simulink model "Control_Logic_e"  (R2021a)
settings: Solver=FixedStepAuto  StartTime=Start_time  StopTime=Stop_time  FixedStep=Sample_time  RelTol=1e-3
undefined symbols (not defined in the file or in its folder): Aset_N1, Aset_N10, Aset_N11, Aset_N12, Aset_N2, Aset_N3, Aset_N4, Aset_N5, Aset_N6, Aset_N7, Aset_N8, Aset_N9, Dset_N1, Dset_N2, Sample_time
(part 3 of 3)

== matlab function Control_Logic_e/OSHOTC8/OSHOTC ==
  data: u input; y output; old input; w_old input
% ワンショット タイマ
%  xがOFFからONに変化してからパラメータで設定した[sec]の間、yをONとする。
%  なお、xのON状態がパラメータで設定した[sec]以上継続した場合、あるいは設定以下
%  しか継続しない場合でも、yのON状態の期間はパラメータで設定した時間となる。
%       ud(1) = u(1) ;:入力信号
%       yold = u(2) ;:前回値
%       set = u(3) ;:時定数
%       timc(1) = u(4) ;:計算刻み
%       timc(2) = u(5) ;:経過時間
%       y : 出力信号
function y  = OSHOTC(u,old,w_old)
       y = zeros(2,1);
       ud1 = logical(u(1));
       yold = logical(old(1));
       set = u(2);
       timc1 = u(3);
       timc2 = w_old(1);
       
    if (ud1 == false) && (yold == false)
        w = 0;
        temp = false;
    else
        if set > timc2
            temp = true;
            w = timc2 + timc1;
        else
            temp = false;
            w = timc2;
            if ud1 == false
                w = 0;
            end
        end
    end
    y(1) = double(temp);
    y(2) = w;
end

== matlab function Control_Logic_e/OSHOTC11/OSHOTC ==
  data: u input; y output; old input; w_old input
% ワンショット タイマ
%  xがOFFからONに変化してからパラメータで設定した[sec]の間、yをONとする。
%  なお、xのON状態がパラメータで設定した[sec]以上継続した場合、あるいは設定以下
%  しか継続しない場合でも、yのON状態の期間はパラメータで設定した時間となる。
%       ud(1) = u(1) ;:入力信号
%       yold = u(2) ;:前回値
%       set = u(3) ;:時定数
%       timc(1) = u(4) ;:計算刻み
%       timc(2) = u(5) ;:経過時間
%       y : 出力信号
function y  = OSHOTC(u,old,w_old)
       y = zeros(2,1);
       ud1 = logical(u(1));
       yold = logical(old(1));
       set = u(2);
       timc1 = u(3);
       timc2 = w_old(1);
       
    if (ud1 == false) && (yold == false)
        w = 0;
        temp = false;
    else
        if set > timc2
            temp = true;
            w = timc2 + timc1;
        else
            temp = false;
            w = timc2;
            if ud1 == false
                w = 0;
            end
        end
    end
    y(1) = double(temp);
    y(2) = w;
end

== matlab function Control_Logic_e/OSHOTC13/OSHOTC ==
  data: u input; y output; old input; w_old input
% ワンショット タイマ
%  xがOFFからONに変化してからパラメータで設定した[sec]の間、yをONとする。
%  なお、xのON状態がパラメータで設定した[sec]以上継続した場合、あるいは設定以下
%  しか継続しない場合でも、yのON状態の期間はパラメータで設定した時間となる。
%       ud(1) = u(1) ;:入力信号
%       yold = u(2) ;:前回値
%       set = u(3) ;:時定数
%       timc(1) = u(4) ;:計算刻み
%       timc(2) = u(5) ;:経過時間
%       y : 出力信号
function y  = OSHOTC(u,old,w_old)
       y = zeros(2,1);
       ud1 = logical(u(1));
       yold = logical(old(1));
       set = u(2);
       timc1 = u(3);
       timc2 = w_old(1);
       
    if (ud1 == false) && (yold == false)
        w = 0;
        temp = false;
    else
        if set > timc2
            temp = true;
            w = timc2 + timc1;
        else
            temp = false;
            w = timc2;
            if ud1 == false
                w = 0;
            end
        end
    end
    y(1) = double(temp);
    y(2) = w;
end

== matlab function Control_Logic_e/NOT4/NOT ==
  data: u input; y output
%反転
function y  = NOT(u)
    y = 0;
    ud = logical(u(1));
    if ud == false        
        temp = true;
    else
        temp = false;
    end
    y = double(temp);
end

== matlab function Control_Logic_e/OSHOTC6/OSHOTC ==
  data: u input; y output; old input; w_old input
% ワンショット タイマ
%  xがOFFからONに変化してからパラメータで設定した[sec]の間、yをONとする。
%  なお、xのON状態がパラメータで設定した[sec]以上継続した場合、あるいは設定以下
%  しか継続しない場合でも、yのON状態の期間はパラメータで設定した時間となる。
%       ud(1) = u(1) ;:入力信号
%       yold = u(2) ;:前回値
%       set = u(3) ;:時定数
%       timc(1) = u(4) ;:計算刻み
%       timc(2) = u(5) ;:経過時間
%       y : 出力信号
function y  = OSHOTC(u,old,w_old)
       y = zeros(2,1);
       ud1 = logical(u(1));
       yold = logical(old(1));
       set = u(2);
       timc1 = u(3);
       timc2 = w_old(1);
       
    if (ud1 == false) && (yold == false)
        w = 0;
        temp = false;
    else
        if set > timc2
            temp = true;
            w = timc2 + timc1;
        else
            temp = false;
            w = timc2;
            if ud1 == false
                w = 0;
            end
        end
    end
    y(1) = double(temp);
    y(2) = w;
end

== matlab function Control_Logic_e/OSHOTC7/OSHOTC ==
  data: u input; y output; old input; w_old input
% ワンショット タイマ
%  xがOFFからONに変化してからパラメータで設定した[sec]の間、yをONとする。
%  なお、xのON状態がパラメータで設定した[sec]以上継続した場合、あるいは設定以下
%  しか継続しない場合でも、yのON状態の期間はパラメータで設定した時間となる。
%       ud(1) = u(1) ;:入力信号
%       yold = u(2) ;:前回値
%       set = u(3) ;:時定数
%       timc(1) = u(4) ;:計算刻み
%       timc(2) = u(5) ;:経過時間
%       y : 出力信号
function y  = OSHOTC(u,old,w_old)
       y = zeros(2,1);
       ud1 = logical(u(1));
       yold = logical(old(1));
       set = u(2);
       timc1 = u(3);
       timc2 = w_old(1);
       
    if (ud1 == false) && (yold == false)
        w = 0;
        temp = false;
    else
        if set > timc2
            temp = true;
            w = timc2 + timc1;
        else
            temp = false;
            w = timc2;
            if ud1 == false
                w = 0;
            end
        end
    end
    y(1) = double(temp);
    y(2) = w;
end

== matlab function Control_Logic_e/OSHOTC14/OSHOTC ==
  data: u input; y output; old input; w_old input
% ワンショット タイマ
%  xがOFFからONに変化してからパラメータで設定した[sec]の間、yをONとする。
%  なお、xのON状態がパラメータで設定した[sec]以上継続した場合、あるいは設定以下
%  しか継続しない場合でも、yのON状態の期間はパラメータで設定した時間となる。
%       ud(1) = u(1) ;:入力信号
%       yold = u(2) ;:前回値
%       set = u(3) ;:時定数
%       timc(1) = u(4) ;:計算刻み
%       timc(2) = u(5) ;:経過時間
%       y : 出力信号
function y  = OSHOTC(u,old,w_old)
       y = zeros(2,1);
       ud1 = logical(u(1));
       yold = logical(old(1));
       set = u(2);
       timc1 = u(3);
       timc2 = w_old(1);
       
    if (ud1 == false) && (yold == false)
        w = 0;
        temp = false;
    else
        if set > timc2
            temp = true;
            w = timc2 + timc1;
        else
            temp = false;
            w = timc2;
            if ud1 == false
                w = 0;
            end
        end
    end
    y(1) = double(temp);
    y(2) = w;
end

== matlab function Control_Logic_e/OR4/MATLAB Function ==
  data: u input; y output
% 論理積
function y  = OR(u)
   y= 0;
   dy = false;
   for i = 1:size(u,1)
   dy = logical(u(i)) | dy;
   end
    y = double(dy);
end

== matlab function Control_Logic_e/OR3/MATLAB Function ==
  data: u input; y output
% 論理積
function y  = OR(u)
   y= 0;
   dy = false;
   for i = 1:size(u,1)
   dy = logical(u(i)) | dy;
   end
    y = double(dy);
end

== matlab function Control_Logic_e/OR5/MATLAB Function ==
  data: u input; y output
% 論理積
function y  = OR(u)
   y= 0;
   dy = false;
   for i = 1:size(u,1)
   dy = logical(u(i)) | dy;
   end
    y = double(dy);
end

== matlab function Control_Logic_e/OR6/MATLAB Function ==
  data: u input; y output
% 論理積
function y  = OR(u)
   y= 0;
   dy = false;
   for i = 1:size(u,1)
   dy = logical(u(i)) | dy;
   end
    y = double(dy);
end

== matlab function Control_Logic_e/OR/MATLAB Function ==
  data: u input; y output
% 論理積
function y  = OR(u)
   y= 0;
   dy = false;
   for i = 1:size(u,1)
   dy = logical(u(i)) | dy;
   end
    y = double(dy);
end

== matlab function Control_Logic_e/OR8/MATLAB Function ==
  data: u input; y output
% 論理積
function y  = OR(u)
   y= 0;
   dy = false;
   for i = 1:size(u,1)
   dy = logical(u(i)) | dy;
   end
    y = double(dy);
end

== matlab function Control_Logic_e/NOT5/NOT ==
  data: u input; y output
%反転
function y  = NOT(u)
    y = 0;
    ud = logical(u(1));
    if ud == false        
        temp = true;
    else
        temp = false;
    end
    y = double(temp);
end

== matlab function Control_Logic_e/OR9/MATLAB Function ==
  data: u input; y output
% 論理積
function y  = OR(u)
   y= 0;
   dy = false;
   for i = 1:size(u,1)
   dy = logical(u(i)) | dy;
   end
    y = double(dy);
end

== matlab function Control_Logic_e/OR7/MATLAB Function ==
  data: u input; y output
% 論理積
function y  = OR(u)
   y= 0;
   dy = false;
   for i = 1:size(u,1)
   dy = logical(u(i)) | dy;
   end
    y = double(dy);
end

== matlab function Control_Logic_e/OR1/MATLAB Function ==
  data: u input; y output
% 論理積
function y  = OR(u)
   y= 0;
   dy = false;
   for i = 1:size(u,1)
   dy = logical(u(i)) | dy;
   end
    y = double(dy);
end

== matlab function Control_Logic_e/ANSW6/MATLAB Function ==
  data: u input; y output
% 2位置(アナログ)スイッチ
%   u3入力がONならば、 y=x1(A入力を選択)
%   u3入力がOFFならば、 y=x2(B入力を選択)
%       u(2):A入力変数
%       u(3):B入力変数
%       u3=u(1):C入力変数
%       y : 出力変数
function y  = ANSW(u)
    y = 0;
    temp = logical(u(1));
    temp2 = 0;
    if temp ~= false
        temp2 = u(2);
    else
        temp2 = u(3); 
    end
    y = temp2;
end

== matlab function Control_Logic_e/LAG/LAG ==
  data: u input; y output; old input
%% lag 1次遅れ
%   function:		PLAG
%    description:	一次遅れ
%	y=(dt×x+τ×yold)/(dt+τ)
%	dt：時間刻み，τ：時定数，yold：前回出力値
%
%    algorithm:
%	if(init == TRUE)	then
%		AY = Y_old = AX
%	endif
%	AY = (dt*AX+τ*Y_old)/(dt+ τ)
%	Y_old = AY

function y  = LAG(u,old)
  y = 0;
  x = u(1);
  tau = u(2);
  dt = u(3);
  y_old = old(1);
  y = (dt*x+tau*y_old)/(dt+ tau);
end

== matlab function Control_Logic_e/LAG1/LAG ==
  data: u input; y output; old input
%% lag 1次遅れ
%   function:		PLAG
%    description:	一次遅れ
%	y=(dt×x+τ×yold)/(dt+τ)
%	dt：時間刻み，τ：時定数，yold：前回出力値
%
%    algorithm:
%	if(init == TRUE)	then
%		AY = Y_old = AX
%	endif
%	AY = (dt*AX+τ*Y_old)/(dt+ τ)
%	Y_old = AY

function y  = LAG(u,old)
  y = 0;
  x = u(1);
  tau = u(2);
  dt = u(3);
  y_old = old(1);
  y = (dt*x+tau*y_old)/(dt+ tau);
end

== matlab function Control_Logic_e/LAG2/LAG ==
  data: u input; y output; old input
%% lag 1次遅れ
%   function:		PLAG
%    description:	一次遅れ
%	y=(dt×x+τ×yold)/(dt+τ)
%	dt：時間刻み，τ：時定数，yold：前回出力値
%
%    algorithm:
%	if(init == TRUE)	then
%		AY = Y_old = AX
%	endif
%	AY = (dt*AX+τ*Y_old)/(dt+ τ)
%	Y_old = AY

function y  = LAG(u,old)
  y = 0;
  x = u(1);
  tau = u(2);
  dt = u(3);
  y_old = old(1);
  y = (dt*x+tau*y_old)/(dt+ tau);
end

== matlab function Control_Logic_e/AND15/AND ==
  data: u input; y output
% 論理積
function y  = AND(u)
   y = 0;
   dy = true;
   for i = 1:size(u,1)
    dy = logical(u(i)) & dy;
   end
    y = double(dy);
end

== matlab function Control_Logic_e/Position control/BRLMT/BRLMT ==
  data: u input; y output; old input
% レートリミッタ
%   |(x-yold)/dt|＜変化レートならば、 y=x
%   |(x-yold)/dt|≧変化レートならば、 y=yold+変化レート
%       u(1)：入力変数
%       yold=u(2)：前回出力値
%       set(1)=u(3)：変化レート
%       set(2)=u(4)：計算刻み
%       y : 出力変数
function y  = BRLMT(u,old)
    y = 0;
    yold = old(1);
    set1= u(2);
    set2= u(3);
    delta = (u(1) - yold) / set2;
    if (delta < set1) && (delta > -set1)
        temp = u(1);
    else
        if delta >= 0 
            temp = yold + set1 * set2;
        else
            temp = yold - set1 * set2;
        end
    end
    y = temp;
end

== matlab function Control_Logic_e/COMP/COMP ==
  data: u input; y output
% 設定値比較
%   x≧Setならば、 yをON
%   x＜Setならば、 yをOFF
%       u=u(1) : 入力変数
%       Set=u(2) : 入力変数
%       y : 出力変数
function y  = COMP(u)
    y = 0;
    set = u(2);
    if u(1) >= set
        temp = true;
    else
        temp = false; 
    end
    y = double(temp);
end

== matlab function Control_Logic_e/Position control/DIV/DIV ==
  data: u input; y output
% 除算器
%       u(1), u(2) : 入力変数
%       set=u(3) : FloatMax
%       y : 出力変数
function y  = DIV(u)
    y = 0;
    temp = double(u(2));
    set = u(3);
    err = -1;
    if temp ~= 0
        y = u(1) / u(2);
    else
        y = set; 
    end
end

== matlab function Control_Logic_e/Position control/DIV2/DIV ==
  data: u input; y output
% 除算器
%       u(1), u(2) : 入力変数
%       set=u(3) : FloatMax
%       y : 出力変数
function y  = DIV(u)
    y = 0;
    temp = double(u(2));
    set = u(3);
    err = -1;
    if temp ~= 0
        y = u(1) / u(2);
    else
        y = set; 
    end
end

== matlab function Control_Logic_e/Position control/HSS/HSS ==
  data: u input; y output
% 高値選択器
function y  = HSS(u)
    y = 0;
    Fmax = u(1);
    for i = 1:size(u,1)
        if u(i) >= Fmax
            Fmax = u(i);
        end 
    end
    y = Fmax;
end

== matlab function Control_Logic_e/Position control/LSS/LSS ==
  data: u input; y output
% 低値選択器
function y  = LSS(u)
    y = 0;
    Fmin = u(1);
    for i = 1:size(u,1)
        if u(i) <= Fmin
            Fmin = u(i);
        end 
    end
    y = Fmin;
end

== matlab function Control_Logic_e/Position control/MUL/MUL ==
  data: u input; y output
% 積算器
function y = MUL(u)
    y = 0;
    temp = 1;
    for i = 1: size(u,1)
        temp = u(i) * temp;
    end
    y = temp;
end

== matlab function Control_Logic_e/Position control/MUL1/MUL ==
  data: u input; y output
% 積算器
function y = MUL(u)
    y = 0;
    temp = 1;
    for i = 1: size(u,1)
        temp = u(i) * temp;
    end
    y = temp;
end

== matlab function Control_Logic_e/Position control/PI/PI ==
  data: u input; y output; old input
% 積分
%   y=Sxdt
%   リセット入力がONのとき、yはリセット値
%       ua：=u(1);% :入力
%       ud=u(2);%：リセット入力
%       yold=u(3);%：前回値
%       set=u(4);%：リセット値
%       timc=u(5);%：計算刻み　dt
function y  = PI(u,old)
       y = 0;
       ua = u(1);% :入力
       ud=logical(u(2));%：リセット入力
       yold=old(1);%：前回値
       set=u(3);%：リセット値
       timc=u(4);%：計算刻み　dt

    if ud == true
        temp = set;
    else
        temp = yold + ua * timc;
    end
    y = temp;
end

== matlab function Control_Logic_e/Position control/SUB/SUB ==
  data: u input; y output
% 減算器
function y = SUB(u)
    y = 0;
    y = u(1) - u(2);
end

== matlab function Control_Logic_e/Position control/SUB1/SUB ==
  data: u input; y output
% 減算器
function y = SUB(u)
    y = 0;
    y = u(1) - u(2);
end

== matlab function Control_Logic_e/Position control/SUB3/SUB ==
  data: u input; y output
% 減算器
function y = SUB(u)
    y = 0;
    y = u(1) - u(2);
end

== matlab function Control_Logic_e/OSHOTC15/OSHOTC ==
  data: u input; y output; old input; w_old input
% ワンショット タイマ
%  xがOFFからONに変化してからパラメータで設定した[sec]の間、yをONとする。
%  なお、xのON状態がパラメータで設定した[sec]以上継続した場合、あるいは設定以下
%  しか継続しない場合でも、yのON状態の期間はパラメータで設定した時間となる。
%       ud(1) = u(1) ;:入力信号
%       yold = u(2) ;:前回値
%       set = u(3) ;:時定数
%       timc(1) = u(4) ;:計算刻み
%       timc(2) = u(5) ;:経過時間
%       y : 出力信号
function y  = OSHOTC(u,old,w_old)
       y = zeros(2,1);
       ud1 = logical(u(1));
       yold = logical(old(1));
       set = u(2);
       timc1 = u(3);
       timc2 = w_old(1);
       
    if (ud1 == false) && (yold == false)
        w = 0;
        temp = false;
    else
        if set > timc2
            temp = true;
            w = timc2 + timc1;
        else
            temp = false;
            w = timc2;
            if ud1 == false
                w = 0;
            end
        end
    end
    y(1) = double(temp);
    y(2) = w;
end

== matlab function Control_Logic_e/Position control/SUM1/SUM ==
  data: u input; y output
% 加算器
function y = SUM(u)
    y = 0;
    temp = 0;
    for i = 1: size(u,1)
        temp = u(i) + temp;
    end
    y = temp;
end

== matlab function Control_Logic_e/Velocity control1/BRLMT/BRLMT ==
  data: u input; y output; old input
% レートリミッタ
%   |(x-yold)/dt|＜変化レートならば、 y=x
%   |(x-yold)/dt|≧変化レートならば、 y=yold+変化レート
%       u(1)：入力変数
%       yold=u(2)：前回出力値
%       set(1)=u(3)：変化レート
%       set(2)=u(4)：計算刻み
%       y : 出力変数
function y  = BRLMT(u,old)
    y = 0;
    yold = old(1);
    set1= u(2);
    set2= u(3);
    delta = (u(1) - yold) / set2;
    if (delta < set1) && (delta > -set1)
        temp = u(1);
    else
        if delta >= 0 
            temp = yold + set1 * set2;
        else
            temp = yold - set1 * set2;
        end
    end
    y = temp;
end

== matlab function Control_Logic_e/Velocity control1/DIV/DIV ==
  data: u input; y output
% 除算器
%       u(1), u(2) : 入力変数
%       set=u(3) : FloatMax
%       y : 出力変数
function y  = DIV(u)
    y = 0;
    temp = double(u(2));
    set = u(3);
    err = -1;
    if temp ~= 0
        y = u(1) / u(2);
    else
        y = set; 
    end
end

== matlab function Control_Logic_e/Velocity control1/DIV2/DIV ==
  data: u input; y output
% 除算器
%       u(1), u(2) : 入力変数
%       set=u(3) : FloatMax
%       y : 出力変数
function y  = DIV(u)
    y = 0;
    temp = double(u(2));
    set = u(3);
    err = -1;
    if temp ~= 0
        y = u(1) / u(2);
    else
        y = set; 
    end
end

== matlab function Control_Logic_e/Velocity control1/HSS/HSS ==
  data: u input; y output
% 高値選択器
function y  = HSS(u)
    y = 0;
    Fmax = u(1);
    for i = 1:size(u,1)
        if u(i) >= Fmax
            Fmax = u(i);
        end 
    end
    y = Fmax;
end

== matlab function Control_Logic_e/Velocity control1/LSS/LSS ==
  data: u input; y output
% 低値選択器
function y  = LSS(u)
    y = 0;
    Fmin = u(1);
    for i = 1:size(u,1)
        if u(i) <= Fmin
            Fmin = u(i);
        end 
    end
    y = Fmin;
end

== matlab function Control_Logic_e/Velocity control1/MUL/MUL ==
  data: u input; y output
% 積算器
function y = MUL(u)
    y = 0;
    temp = 1;
    for i = 1: size(u,1)
        temp = u(i) * temp;
    end
    y = temp;
end

== matlab function Control_Logic_e/Velocity control1/MUL1/MUL ==
  data: u input; y output
% 積算器
function y = MUL(u)
    y = 0;
    temp = 1;
    for i = 1: size(u,1)
        temp = u(i) * temp;
    end
    y = temp;
end

== matlab function Control_Logic_e/Velocity control1/PI/PI ==
  data: u input; y output; old input
% 積分
%   y=Sxdt
%   リセット入力がONのとき、yはリセット値
%       ua：=u(1);% :入力
%       ud=u(2);%：リセット入力
%       yold=u(3);%：前回値
%       set=u(4);%：リセット値
%       timc=u(5);%：計算刻み　dt
function y  = PI(u,old)
       y = 0;
       ua = u(1);% :入力
       ud=logical(u(2));%：リセット入力
       yold=old(1);%：前回値
       set=u(3);%：リセット値
       timc=u(4);%：計算刻み　dt

    if ud == true
        temp = set;
    else
        temp = yold + ua * timc;
    end
    y = temp;
end

== matlab function Control_Logic_e/Velocity control1/SUB/SUB ==
  data: u input; y output
% 減算器
function y = SUB(u)
    y = 0;
    y = u(1) - u(2);
end

== matlab function Control_Logic_e/Velocity control1/SUB1/SUB ==
  data: u input; y output
% 減算器
function y = SUB(u)
    y = 0;
    y = u(1) - u(2);
end

== matlab function Control_Logic_e/Velocity control1/SUB3/SUB ==
  data: u input; y output
% 減算器
function y = SUB(u)
    y = 0;
    y = u(1) - u(2);
end

== matlab function Control_Logic_e/Velocity control1/SUM1/SUM ==
  data: u input; y output
% 加算器
function y = SUM(u)
    y = 0;
    temp = 0;
    for i = 1: size(u,1)
        temp = u(i) + temp;
    end
    y = temp;
end

== matlab function Control_Logic_e/ONDLC/ONDLC ==
  data: u input; y output; old input
% オンディレイ タイマ
%  xがONとなってからパラメータで設定した[sec]後にyがONとなる。
%  なお、xのON状態がパラメータで設定した[sec]続かずにOFF状態
%  へ戻った場合はyはOFF状態を継続する。
%       ud=u(1) :入力信号
%       set=u(2)：時定数
%       timc(1)=u(3)：計算刻み
%       timc(2)=u(4)：経過時間(前回値)
%       y : 出力信号
function y  = ONDLC(u, old)
       y=zeros(2,1);
       ud = logical(u(1));
       set=u(2);
       timc1=u(3);
       timc2=old(1);
    if ud == false
        temp = false;
        w = 0;
    else
        if timc2 < set 
            temp = false;
            w = timc2 + timc1;
        else
            temp = true;
            w = timc2;
        end
    end
    
    y(1)=double(temp);
    y(2)=w;
end

== matlab function Control_Logic_e/SUB/SUB ==
  data: u input; y output
% 減算器
function y = SUB(u)
    y = 0;
    y = u(1) - u(2);
end

== matlab function Control_Logic_e/ONDLC1/ONDLC ==
  data: u input; y output; old input
% オンディレイ タイマ
%  xがONとなってからパラメータで設定した[sec]後にyがONとなる。
%  なお、xのON状態がパラメータで設定した[sec]続かずにOFF状態
%  へ戻った場合はyはOFF状態を継続する。
%       ud=u(1) :入力信号
%       set=u(2)：時定数
%       timc(1)=u(3)：計算刻み
%       timc(2)=u(4)：経過時間(前回値)
%       y : 出力信号
function y  = ONDLC(u, old)
       y=zeros(2,1);
       ud = logical(u(1));
       set=u(2);
       timc1=u(3);
       timc2=old(1);
    if ud == false
        temp = false;
        w = 0;
    else
        if timc2 < set 
            temp = false;
            w = timc2 + timc1;
        else
            temp = true;
            w = timc2;
        end
    end
    
    y(1)=double(temp);
    y(2)=w;
end

== matlab function Control_Logic_e/NOT6/NOT ==
  data: u input; y output
%反転
function y  = NOT(u)
    y = 0;
    ud = logical(u(1));
    if ud == false        
        temp = true;
    else
        temp = false;
    end
    y = double(temp);
end
